simulink model "Comparison_between_Controllers_Ideal_PID_Form"  (R2018b)
settings: Solver=VariableStepAuto  StartTime=0.0  StopTime=500  FixedStep=1  RelTol=1e-3
undefined symbols (not defined in the file or in its folder): idss, s
libraries: cstblocks x29, simulink x14, peGeneralControl x4, slident x4, mpclib x3
(part 1 of 2)
settings Model: Creator=Trips  LastModifiedBy=Trips

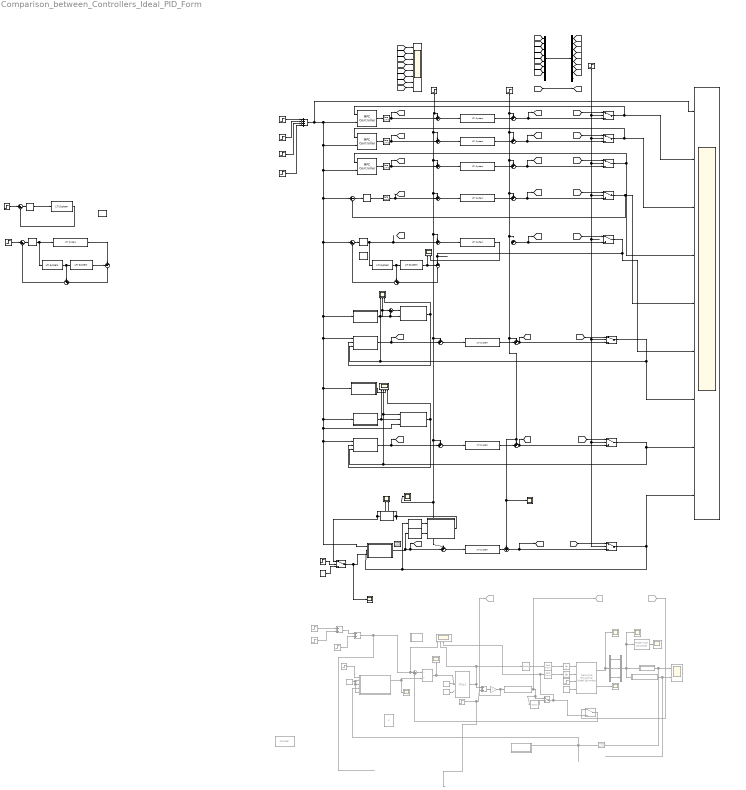
== system Comparison_between_Controllers_Ideal_PID_Form ==
  note: Winner Winner Chicken Dinner!
  note: MPC
  note: Testbedingungen: verändern der Totzeit und verändern der Verstärkung
  note: PI
  note: Smith Predictor
  note: Z
  note: Uncertainties
  note: Plant
  note: MRAC
  note: Z
  note: MIAC
  note: MRAC Better
  note: offset wegrechnen...
  Adaptive Mechanism : Subsystem
  Adaptive Mechanism1 : Subsystem
  Adaptive PI Controller : Subsystem  Commented=on
  Adaptive SmithPredictor : Subsystem
  Adaptive SmithPredictor1 : Subsystem
  Adaptive SmithPredictor2 : Subsystem
  Add{,1..9,11..12,16..17} (14 alike) : Sum  Inputs=++|
  Add10 : Sum  Inputs=++++
  Add13 : Sum  Commented=on
  Add14 : Sum  Commented=on
  Add15 : Sum  Commented=on
  Bus Creator2 : BusCreator  Commented=on  Inputs=3
  Bus Selector2 : BusSelector  Commented=on  OutputSignals=A,B,Ts
  Calculate DC Gain : Subsystem  Commented=on
  Calculate Time Constant : Subsystem  Commented=on
  Chien Hrones Reswick : Subsystem  Commented=on
  Constant1 : Constant  Value=0.5
  Constant6 : Constant  Commented=on  Value=0
  Demux : Demux  Outputs=8
  Divide1 : Product  Commented=on  Inputs=*/  OutMin=[1]  OutMax=[1]
  From24 : From  Commented=on  GotoTag=B8
  Gain1 : Gain  Commented=on
  Goto24 : Goto  Commented=on  GotoTag=U8
  Goto25 : Goto  Commented=on  GotoTag=A8
  Idmodel : slident/Models/Idmodel  Commented=on  sys=idss(-1,1,1,0,'Ts',1)  IC=0  noi=on  seed=[]
      settings: SourceProductName=System Identification Toolbox  SourceProductBaseCode=ID
  Kp_init : Constant  Commented=on
  Kp_init1 : Constant  Commented=on
  LTI System1 : cstblocks/LTI System  sys=0.5/(700*s+1)  IC=[]
  LTI System16 : cstblocks/LTI System  sys=0.5/(700*s+1)  IC=[]
  LTI System17 : cstblocks/LTI System  sys=exp(-s*600)  IC=[]
  LTI System2 : cstblocks/LTI System  sys=exp(-s*600)  IC=[]
  LTI System3 : cstblocks/LTI System  sys=0.5/(700*s+1)  IC=[]
  Low-Pass Filter (Discrete or Continuous) : peGeneralControl/Low-Pass Filter (Discrete or Continuous)  K=1  T=1200  B=inf  A=-inf  Ts=-1
  Low-Pass Filter (Discrete or Continuous)1 : peGeneralControl/Low-Pass Filter (Discrete or Continuous)  K=1  T=1200  B=inf  A=-inf  Ts=-1
  Low-Pass Filter (Discrete or Continuous)2 : peGeneralControl/Low-Pass Filter (Discrete or Continuous)  K=1  T=1200  B=inf  A=-inf  Ts=-1
  MPCFast_Robust : mpclib/MPC Controller  SCDEnableBlockLinearizationSpecification=on  mpcobj=mpc1_Faster_Robust  is_multiple=0  enable_value=0  return_u0=off  updateMPCinCallerWorkspace=on  md_inport=off  mv_inport=off  return_cost=off  return_mvseq=off  return_qpstatus=off  return_xseq=off  return_state=off  return_ovseq=off  state_inport=off  umin_inport=off  umax_inport=off  ymin_inport=off  ymax_inport=off  cc_inport=off  ywt_inport=off  uwt_inport=off  duwt_inport=off  rhoeps_inport=off  uref_inport=off  n_ts=70  n_p=15  n_mv=1  n_md=0  n_ud=0  n_mo=1  n_uo=0  BlockDataType=double  SampleTimeInherited=off  switch_inport=off
  MPCStandard : mpclib/MPC Controller  SCDEnableBlockLinearizationSpecification=on  mpcobj=mpc_Standard  is_multiple=0  enable_value=0  return_u0=off  updateMPCinCallerWorkspace=on  md_inport=off  mv_inport=off  return_cost=off  return_mvseq=off  return_qpstatus=off  return_xseq=off  return_state=off  return_ovseq=off  state_inport=off  umin_inport=off  umax_inport=off  ymin_inport=off  ymax_inport=off  cc_inport=off  ywt_inport=off  uwt_inport=off  duwt_inport=off  rhoeps_inport=off  uref_inport=off  n_ts=153  n_p=10  n_mv=1  n_md=0  n_ud=0  n_mo=1  n_uo=0  BlockDataType=double  SampleTimeInherited=off  switch_inport=off
  MPCStandardRobust : mpclib/MPC Controller  SCDEnableBlockLinearizationSpecification=on  mpcobj=mpc1_Standard_Robust  is_multiple=0  enable_value=0  return_u0=off  updateMPCinCallerWorkspace=on  md_inport=off  mv_inport=off  return_cost=off  return_mvseq=off  return_qpstatus=off  return_xseq=off  return_state=off  return_ovseq=off  state_inport=off  umin_inport=off  umax_inport=off  ymin_inport=off  ymax_inport=off  cc_inport=off  ywt_inport=off  uwt_inport=off  duwt_inport=off  rhoeps_inport=off  uref_inport=off  n_ts=153  n_p=10  n_mv=1  n_md=0  n_ud=0  n_mo=1  n_uo=0  BlockDataType=double  SampleTimeInherited=off  switch_inport=off
  Manual Switch : ManualSwitch  Commented=on
  Minus : Sum  Inputs=|+-
  Model Type Converter1 : slident/Estimators/Model Type Converter  Commented=on  InputModelType=ARX
      settings: SourceProductName=System Identification Toolbox  SourceProductBaseCode=ID
  Multiply : Product  Commented=on
  Mux : Mux  Inputs=8
  Outputs : Scope  NumInputPorts=9
  PID Controller : simulink/Continuous/PID Controller  Controller=PI  Form=Parallel  TimeDomain=Continuous-time  SampleTime=-1  IntegratorMethod=Forward Euler  FilterMethod=Forward Euler  ControllerParametersSource=internal  P=1.81017492228937  I=0.00195107565412744  D=118.272348286844  UseFilter=on  N=0.00420306193364532  TunerSelectOption=Transfer Function Based (PID Tuner App)  InitialConditionSource=internal  InitialConditionForIntegrator=0  InitialConditionForFilter=0  DifferentiatorICPrevScaledInput=0  ExternalReset=none  TrackingMode=off  Kt=1  LimitOutput=on  UpperSaturationLimit=100  LowerSaturationLimit=0  LinearizeAsGain=on  AntiWindupMode=none  Kb=1  POutMin=[]  POutMax=[]  IOutMin=[]  IOutMax=[]  DOutMin=[]  DOutMax=[]  NOutMin=[]  NOutMax=[]  SumOutMin=[]  SumOutMax=[]  SaturationOutMin=[]  SaturationOutMax=[]  PParamMin=[]  PParamMax=[]  IParamMin=[]  IParamMax=[]  DParamMin=[]  DParamMax=[]  NParamMin=[]  NParamMax=[]  KbParamMin=[]  KbParamMax=[]  KtParamMin=[]  KtParamMax=[]  KbOutMin=[]  KbOutMax=[]  KtOutMin=[]  KtOutMax=[]  IntegratorOutMin=[]  IntegratorOutMax=[]  FilterOutMin=[]  FilterOutMax=[]  SumI1OutMin=[]  SumI1OutMax=[]  SumI2OutMin=[]  SumI2OutMax=[]  SumI3OutMin=[]  SumI3OutMax=[]  SumI4OutMin=[]  SumI4OutMax=[]  SumDOutMin=[]  SumDOutMax=[]  DifferentiatorOutMin=[]  DifferentiatorOutMax=[]  FilterDiffOutCoefMin=[]  FilterDiffOutCoefMax=[]  ReciprocalOutMin=[]  ReciprocalOutMax=[]  SumDenOutMin=[]  SumDenOutMax=[]  SumNumOutMin=[]  SumNumOutMax=[]  DivideOutMin=[]  DivideOutMax=[]  IntegratorContinuousStateAttributes=''  IntegratorStateMustResolveToSignalObject=off  IntegratorRTWStateStorageClass=Auto  FilterContinuousStateAttributes=''  FilterStateMustResolveToSignalObject=off  FilterRTWStateStorageClass=Auto  ParallelPVariant=InternalParameters  IdealPVariant=Disabled  IVariant=InternalParameters  DVariant=Disabled  IntegratorVariant=Continuous  SatVariant=Enabled  AWVariant=Passthrough  PCopyVariant=Disabled  TRVariant=Disabled  FdbkBlocksVariant=Forward  IdealPFdbkVariant=Disabled  SatFdbkVariant=Disabled  DerivativeFilterVariant=Disabled  NVariant=Disabled  NCopyVariant=Disabled_SignalSpec  FilterICVariant=Disabled  IntegratorICVariant=InternalICs  ExternalResetVariant=Disabled  TRSumVariant=Passthrough  SumFdbkVariant=Disabled  SumVariant=Sum_PI
  PID Controller1 : simulink/Continuous/PID Controller  Controller=PI  Form=Parallel  TimeDomain=Continuous-time  SampleTime=-1  IntegratorMethod=Forward Euler  FilterMethod=Forward Euler  ControllerParametersSource=internal  P=2.08480938092905  I=0.0089383224092643  D=118.272348286844  UseFilter=on  N=0.00420306193364532  TunerSelectOption=Transfer Function Based (PID Tuner App)  InitialConditionSource=internal  InitialConditionForIntegrator=0  InitialConditionForFilter=0  DifferentiatorICPrevScaledInput=0  ExternalReset=none  TrackingMode=off  Kt=1  LimitOutput=on  UpperSaturationLimit=100  LowerSaturationLimit=0  LinearizeAsGain=on  AntiWindupMode=none  Kb=1  POutMin=[]  POutMax=[]  IOutMin=[]  IOutMax=[]  DOutMin=[]  DOutMax=[]  NOutMin=[]  NOutMax=[]  SumOutMin=[]  SumOutMax=[]  SaturationOutMin=[]  SaturationOutMax=[]  PParamMin=[]  PParamMax=[]  IParamMin=[]  IParamMax=[]  DParamMin=[]  DParamMax=[]  NParamMin=[]  NParamMax=[]  KbParamMin=[]  KbParamMax=[]  KtParamMin=[]  KtParamMax=[]  KbOutMin=[]  KbOutMax=[]  KtOutMin=[]  KtOutMax=[]  IntegratorOutMin=[]  IntegratorOutMax=[]  FilterOutMin=[]  FilterOutMax=[]  SumI1OutMin=[]  SumI1OutMax=[]  SumI2OutMin=[]  SumI2OutMax=[]  SumI3OutMin=[]  SumI3OutMax=[]  SumI4OutMin=[]  SumI4OutMax=[]  SumDOutMin=[]  SumDOutMax=[]  DifferentiatorOutMin=[]  DifferentiatorOutMax=[]  FilterDiffOutCoefMin=[]  FilterDiffOutCoefMax=[]  ReciprocalOutMin=[]  ReciprocalOutMax=[]  SumDenOutMin=[]  SumDenOutMax=[]  SumNumOutMin=[]  SumNumOutMax=[]  DivideOutMin=[]  DivideOutMax=[]  IntegratorContinuousStateAttributes=''  IntegratorStateMustResolveToSignalObject=off  IntegratorRTWStateStorageClass=Auto  FilterContinuousStateAttributes=''  FilterStateMustResolveToSignalObject=off  FilterRTWStateStorageClass=Auto  ParallelPVariant=InternalParameters  IdealPVariant=Disabled  IVariant=InternalParameters  DVariant=Disabled  IntegratorVariant=Continuous  SatVariant=Enabled  AWVariant=Passthrough  PCopyVariant=Disabled  TRVariant=Disabled  FdbkBlocksVariant=Forward  IdealPFdbkVariant=Disabled  SatFdbkVariant=Disabled  DerivativeFilterVariant=Disabled  NVariant=Disabled  NCopyVariant=Disabled_SignalSpec  FilterICVariant=Disabled  IntegratorICVariant=InternalICs  ExternalResetVariant=Disabled  TRSumVariant=Passthrough  SumFdbkVariant=Disabled  SumVariant=Sum_PI
  PID Controller2 : simulink/Continuous/PID Controller  Controller=PI  Form=Ideal  TimeDomain=Continuous-time  SampleTime=-1  IntegratorMethod=Forward Euler  FilterMethod=Forward Euler  ControllerParametersSource=internal  P=3.04732259067536  I=0.00445689106465138  D=118.272348286844  UseFilter=on  N=0.00420306193364532  TunerSelectOption=Transfer Function Based (PID Tuner App)  InitialConditionSource=internal  InitialConditionForIntegrator=0  InitialConditionForFilter=0  DifferentiatorICPrevScaledInput=0  ExternalReset=none  TrackingMode=off  Kt=1  LimitOutput=on  UpperSaturationLimit=100  LowerSaturationLimit=0  LinearizeAsGain=on  AntiWindupMode=none  Kb=1  POutMin=[]  POutMax=[]  IOutMin=[]  IOutMax=[]  DOutMin=[]  DOutMax=[]  NOutMin=[]  NOutMax=[]  SumOutMin=[]  SumOutMax=[]  SaturationOutMin=[]  SaturationOutMax=[]  PParamMin=[]  PParamMax=[]  IParamMin=[]  IParamMax=[]  DParamMin=[]  DParamMax=[]  NParamMin=[]  NParamMax=[]  KbParamMin=[]  KbParamMax=[]  KtParamMin=[]  KtParamMax=[]  KbOutMin=[]  KbOutMax=[]  KtOutMin=[]  KtOutMax=[]  IntegratorOutMin=[]  IntegratorOutMax=[]  FilterOutMin=[]  FilterOutMax=[]  SumI1OutMin=[]  SumI1OutMax=[]  SumI2OutMin=[]  SumI2OutMax=[]  SumI3OutMin=[]  SumI3OutMax=[]  SumI4OutMin=[]  SumI4OutMax=[]  SumDOutMin=[]  SumDOutMax=[]  DifferentiatorOutMin=[]  DifferentiatorOutMax=[]  FilterDiffOutCoefMin=[]  FilterDiffOutCoefMax=[]  ReciprocalOutMin=[]  ReciprocalOutMax=[]  SumDenOutMin=[]  SumDenOutMax=[]  SumNumOutMin=[]  SumNumOutMax=[]  DivideOutMin=[]  DivideOutMax=[]  IntegratorContinuousStateAttributes=''  IntegratorStateMustResolveToSignalObject=off  IntegratorRTWStateStorageClass=Auto  FilterContinuousStateAttributes=''  FilterStateMustResolveToSignalObject=off  FilterRTWStateStorageClass=Auto  ParallelPVariant=Passthrough  IdealPVariant=InternalParameters  IVariant=InternalParameters  DVariant=Disabled  IntegratorVariant=Continuous  SatVariant=Enabled  AWVariant=Passthrough  PCopyVariant=Disabled  TRVariant=Disabled  FdbkBlocksVariant=Forward  IdealPFdbkVariant=Disabled  SatFdbkVariant=Disabled  DerivativeFilterVariant=Disabled  NVariant=Disabled  NCopyVariant=Disabled_SignalSpec  FilterICVariant=Disabled  IntegratorICVariant=InternalICs  ExternalResetVariant=Disabled  TRSumVariant=Passthrough  SumFdbkVariant=Disabled  SumVariant=Sum_PI
  PID Controller3 : simulink/Continuous/PID Controller  Commented=on  Controller=PI  Form=Ideal  TimeDomain=Continuous-time  SampleTime=-1  IntegratorMethod=Forward Euler  FilterMethod=Forward Euler  ControllerParametersSource=internal  P=1.00442837242696  I=0.00143977155212025  D=0  UseFilter=on  N=100  TunerSelectOption=Transfer Function Based (PID Tuner App)  InitialConditionSource=internal  InitialConditionForIntegrator=0  InitialConditionForFilter=0  DifferentiatorICPrevScaledInput=0  ExternalReset=none  TrackingMode=off  Kt=1  LimitOutput=on  UpperSaturationLimit=100  LowerSaturationLimit=-100  LinearizeAsGain=on  AntiWindupMode=none  Kb=1  POutMin=[]  POutMax=[]  IOutMin=[]  IOutMax=[]  DOutMin=[]  DOutMax=[]  NOutMin=[]  NOutMax=[]  SumOutMin=[]  SumOutMax=[]  SaturationOutMin=[]  SaturationOutMax=[]  PParamMin=[]  PParamMax=[]  IParamMin=[]  IParamMax=[]  DParamMin=[]  DParamMax=[]  NParamMin=[]  NParamMax=[]  KbParamMin=[]  KbParamMax=[]  KtParamMin=[]  KtParamMax=[]  KbOutMin=[]  KbOutMax=[]  KtOutMin=[]  KtOutMax=[]  IntegratorOutMin=[]  IntegratorOutMax=[]  FilterOutMin=[]  FilterOutMax=[]  SumI1OutMin=[]  SumI1OutMax=[]  SumI2OutMin=[]  SumI2OutMax=[]  SumI3OutMin=[]  SumI3OutMax=[]  SumI4OutMin=[]  SumI4OutMax=[]  SumDOutMin=[]  SumDOutMax=[]  DifferentiatorOutMin=[]  DifferentiatorOutMax=[]  FilterDiffOutCoefMin=[]  FilterDiffOutCoefMax=[]  ReciprocalOutMin=[]  ReciprocalOutMax=[]  SumDenOutMin=[]  SumDenOutMax=[]  SumNumOutMin=[]  SumNumOutMax=[]  DivideOutMin=[]  DivideOutMax=[]  IntegratorContinuousStateAttributes=''  IntegratorStateMustResolveToSignalObject=off  IntegratorRTWStateStorageClass=Auto  FilterContinuousStateAttributes=''  FilterStateMustResolveToSignalObject=off  FilterRTWStateStorageClass=Auto  ParallelPVariant=Passthrough  IdealPVariant=InternalParameters  IVariant=InternalParameters  DVariant=Disabled  IntegratorVariant=Continuous  SatVariant=Enabled  AWVariant=Passthrough  PCopyVariant=Disabled  TRVariant=Disabled  FdbkBlocksVariant=Forward  IdealPFdbkVariant=Disabled  SatFdbkVariant=Disabled  DerivativeFilterVariant=Disabled  NVariant=Disabled  NCopyVariant=Disabled_SignalSpec  FilterICVariant=Disabled  IntegratorICVariant=InternalICs  ExternalResetVariant=Disabled  TRSumVariant=Passthrough  SumFdbkVariant=Disabled  SumVariant=Sum_PI
  PID Controller4 : simulink/Continuous/PID Controller  Controller=PID  Form=Parallel  TimeDomain=Continuous-time  SampleTime=-1  IntegratorMethod=Forward Euler  FilterMethod=Forward Euler  ControllerParametersSource=internal  P=1  I=1  D=0  UseFilter=on  N=100  TunerSelectOption=Transfer Function Based (PID Tuner App)  InitialConditionSource=internal  InitialConditionForIntegrator=0  InitialConditionForFilter=0  DifferentiatorICPrevScaledInput=0  ExternalReset=none  TrackingMode=off  Kt=1  LimitOutput=off  UpperSaturationLimit=inf  LowerSaturationLimit=-inf  LinearizeAsGain=on  AntiWindupMode=none  Kb=1  POutMin=[]  POutMax=[]  IOutMin=[]  IOutMax=[]  DOutMin=[]  DOutMax=[]  NOutMin=[]  NOutMax=[]  SumOutMin=[]  SumOutMax=[]  SaturationOutMin=[]  SaturationOutMax=[]  PParamMin=[]  PParamMax=[]  IParamMin=[]  IParamMax=[]  DParamMin=[]  DParamMax=[]  NParamMin=[]  NParamMax=[]  KbParamMin=[]  KbParamMax=[]  KtParamMin=[]  KtParamMax=[]  KbOutMin=[]  KbOutMax=[]  KtOutMin=[]  KtOutMax=[]  IntegratorOutMin=[]  IntegratorOutMax=[]  FilterOutMin=[]  FilterOutMax=[]  SumI1OutMin=[]  SumI1OutMax=[]  SumI2OutMin=[]  SumI2OutMax=[]  SumI3OutMin=[]  SumI3OutMax=[]  SumI4OutMin=[]  SumI4OutMax=[]  SumDOutMin=[]  SumDOutMax=[]  DifferentiatorOutMin=[]  DifferentiatorOutMax=[]  FilterDiffOutCoefMin=[]  FilterDiffOutCoefMax=[]  ReciprocalOutMin=[]  ReciprocalOutMax=[]  SumDenOutMin=[]  SumDenOutMax=[]  SumNumOutMin=[]  SumNumOutMax=[]  DivideOutMin=[]  DivideOutMax=[]  IntegratorContinuousStateAttributes=''  IntegratorStateMustResolveToSignalObject=off  IntegratorRTWStateStorageClass=Auto  FilterContinuousStateAttributes=''  FilterStateMustResolveToSignalObject=off  FilterRTWStateStorageClass=Auto  ParallelPVariant=InternalParameters  IdealPVariant=Disabled  IVariant=InternalParameters  DVariant=InternalParameters  IntegratorVariant=Continuous  SatVariant=Disabled  AWVariant=Passthrough  PCopyVariant=Disabled  TRVariant=Disabled  FdbkBlocksVariant=Forward  IdealPFdbkVariant=Disabled  SatFdbkVariant=Disabled  DerivativeFilterVariant=ContFilter  NVariant=InternalParameters  NCopyVariant=Disabled  FilterICVariant=InternalICsFilter  IntegratorICVariant=InternalICs  ExternalResetVariant=Disabled  TRSumVariant=Passthrough  SumFdbkVariant=Disabled  SumVariant=Sum_PID
  PID Controller5 : simulink/Continuous/PID Controller  Controller=PI  Form=Parallel  TimeDomain=Continuous-time  SampleTime=-1  IntegratorMethod=Forward Euler  FilterMethod=Forward Euler  ControllerParametersSource=internal  P=3.04732259067536  I=0.00445689106465138  D=118.272348286844  UseFilter=on  N=0.00420306193364532  TunerSelectOption=Transfer Function Based (PID Tuner App)  InitialConditionSource=internal  InitialConditionForIntegrator=0  InitialConditionForFilter=0  DifferentiatorICPrevScaledInput=0  ExternalReset=none  TrackingMode=off  Kt=1  LimitOutput=on  UpperSaturationLimit=100  LowerSaturationLimit=0  LinearizeAsGain=on  AntiWindupMode=none  Kb=1  POutMin=[]  POutMax=[]  IOutMin=[]  IOutMax=[]  DOutMin=[]  DOutMax=[]  NOutMin=[]  NOutMax=[]  SumOutMin=[]  SumOutMax=[]  SaturationOutMin=[]  SaturationOutMax=[]  PParamMin=[]  PParamMax=[]  IParamMin=[]  IParamMax=[]  DParamMin=[]  DParamMax=[]  NParamMin=[]  NParamMax=[]  KbParamMin=[]  KbParamMax=[]  KtParamMin=[]  KtParamMax=[]  KbOutMin=[]  KbOutMax=[]  KtOutMin=[]  KtOutMax=[]  IntegratorOutMin=[]  IntegratorOutMax=[]  FilterOutMin=[]  FilterOutMax=[]  SumI1OutMin=[]  SumI1OutMax=[]  SumI2OutMin=[]  SumI2OutMax=[]  SumI3OutMin=[]  SumI3OutMax=[]  SumI4OutMin=[]  SumI4OutMax=[]  SumDOutMin=[]  SumDOutMax=[]  DifferentiatorOutMin=[]  DifferentiatorOutMax=[]  FilterDiffOutCoefMin=[]  FilterDiffOutCoefMax=[]  ReciprocalOutMin=[]  ReciprocalOutMax=[]  SumDenOutMin=[]  SumDenOutMax=[]  SumNumOutMin=[]  SumNumOutMax=[]  DivideOutMin=[]  DivideOutMax=[]  IntegratorContinuousStateAttributes=''  IntegratorStateMustResolveToSignalObject=off  IntegratorRTWStateStorageClass=Auto  FilterContinuousStateAttributes=''  FilterStateMustResolveToSignalObject=off  FilterRTWStateStorageClass=Auto  ParallelPVariant=InternalParameters  IdealPVariant=Disabled  IVariant=InternalParameters  DVariant=Disabled  IntegratorVariant=Continuous  SatVariant=Enabled  AWVariant=Passthrough  PCopyVariant=Disabled  TRVariant=Disabled  FdbkBlocksVariant=Forward  IdealPFdbkVariant=Disabled  SatFdbkVariant=Disabled  DerivativeFilterVariant=Disabled  NVariant=Disabled  NCopyVariant=Disabled_SignalSpec  FilterICVariant=Disabled  IntegratorICVariant=InternalICs  ExternalResetVariant=Disabled  TRSumVariant=Passthrough  SumFdbkVariant=Disabled  SumVariant=Sum_PI
  PID Controller6 : simulink/Continuous/PID Controller  Controller=PI  Form=Parallel  TimeDomain=Continuous-time  SampleTime=-1  IntegratorMethod=Forward Euler  FilterMethod=Forward Euler  ControllerParametersSource=internal  P=1  I=1  D=0  UseFilter=on  N=100  TunerSelectOption=Transfer Function Based (PID Tuner App)  InitialConditionSource=internal  InitialConditionForIntegrator=0  InitialConditionForFilter=0  DifferentiatorICPrevScaledInput=0  ExternalReset=none  TrackingMode=off  Kt=1  LimitOutput=off  UpperSaturationLimit=inf  LowerSaturationLimit=-inf  LinearizeAsGain=on  AntiWindupMode=none  Kb=1  POutMin=[]  POutMax=[]  IOutMin=[]  IOutMax=[]  DOutMin=[]  DOutMax=[]  NOutMin=[]  NOutMax=[]  SumOutMin=[]  SumOutMax=[]  SaturationOutMin=[]  SaturationOutMax=[]  PParamMin=[]  PParamMax=[]  IParamMin=[]  IParamMax=[]  DParamMin=[]  DParamMax=[]  NParamMin=[]  NParamMax=[]  KbParamMin=[]  KbParamMax=[]  KtParamMin=[]  KtParamMax=[]  KbOutMin=[]  KbOutMax=[]  KtOutMin=[]  KtOutMax=[]  IntegratorOutMin=[]  IntegratorOutMax=[]  FilterOutMin=[]  FilterOutMax=[]  SumI1OutMin=[]  SumI1OutMax=[]  SumI2OutMin=[]  SumI2OutMax=[]  SumI3OutMin=[]  SumI3OutMax=[]  SumI4OutMin=[]  SumI4OutMax=[]  SumDOutMin=[]  SumDOutMax=[]  DifferentiatorOutMin=[]  DifferentiatorOutMax=[]  FilterDiffOutCoefMin=[]  FilterDiffOutCoefMax=[]  ReciprocalOutMin=[]  ReciprocalOutMax=[]  SumDenOutMin=[]  SumDenOutMax=[]  SumNumOutMin=[]  SumNumOutMax=[]  DivideOutMin=[]  DivideOutMax=[]  IntegratorContinuousStateAttributes=''  IntegratorStateMustResolveToSignalObject=off  IntegratorRTWStateStorageClass=Auto  FilterContinuousStateAttributes=''  FilterStateMustResolveToSignalObject=off  FilterRTWStateStorageClass=Auto  ParallelPVariant=InternalParameters  IdealPVariant=Disabled  IVariant=InternalParameters  DVariant=Disabled  IntegratorVariant=Continuous  SatVariant=Disabled  AWVariant=Passthrough  PCopyVariant=Disabled  TRVariant=Disabled  FdbkBlocksVariant=Forward  IdealPFdbkVariant=Disabled  SatFdbkVariant=Disabled  DerivativeFilterVariant=Disabled  NVariant=Disabled  NCopyVariant=Disabled_SignalSpec  FilterICVariant=Disabled  IntegratorICVariant=InternalICs  ExternalResetVariant=Disabled  TRSumVariant=Passthrough  SumFdbkVariant=Disabled  SumVariant=Sum_PI
  Plant{,1..7,9} (9 alike) : cstblocks/LTI System  sys=0.5/(700*s+1)*exp(-s*600)  IC=[]
  Plant8 : cstblocks/LTI System  Commented=on  sys=0.5/(700*s+1)*exp(-s*600)  IC=[]
  Rate Limiter{1..2,4..6} (5 alike) : RateLimiter  RisingSlewLimit=0.05  FallingSlewLimit=-0.05  SampleTimeMode=inherited
  Rate Limiter3 : RateLimiter  Commented=on  SampleTimeMode=inherited
  Rate Transition : RateTransition  Commented=on  OutPortSampleTime=10
  Rate Transition1 : RateTransition  Commented=on  OutPortSampleTime=10
  Recursive Polynomial Model Estimator1 : slident/Estimators/Recursive Polynomial Model Estimator  Commented=on  ModelStructure=ARX  InitialEstimateSource=None  A0=1  B0=1  C0=1  D0=1  F0=1  nk=1  P0=1  InitialInputs=0  InitialOutputs=0  History=Infinite  WindowLength=6000  EstimationMethod=Kalman Filter  AdaptationParameter=0.1  HasTimeVaryingAdaptationParameter=off  NormalizationBias=eps  OutputError=on  OutputP=off  AddEnablePort=on  ExternalReset=Rising  InputProcessing=Sample-based  Ts=10
      settings: SourceProductName=System Identification Toolbox  SourceProductBaseCode=ID
  Reference_Model : Subsystem
  Reference_Model1 : Subsystem
  Reference_Model2 : Subsystem
  References : Step
  References1 : Step  Time=12000  After=2
  References2 : Step  Time=18000  After=3
  References3 : Step  Time=35000  After=3
  Scope : Scope  NumInputPorts=8
  Scope1 : Scope  NumInputPorts=2
  Scope10 : Scope  Commented=on  NumInputPorts=2
  Scope{5,7..9,11..12} (6 alike) : Scope  Commented=on
  Scope13 : Scope
  Scope14 : Scope
  Scope15 : Scope
  Scope2 : Scope  NumInputPorts=2
  Scope3 : Scope  NumInputPorts=4
  Scope4 : Scope  NumInputPorts=3
  Scope6 : Scope  Commented=on  NumInputPorts=5
  Starte adaption : Step  Commented=on  Time=0  SampleTime=1
  Step : Step  Time=0  SampleTime=1
  Step1 : Step  Time=4000  After=0  SampleTime=0
  Step10 : Step  SampleTime=0
  Step2 : Step  Time=4000  SampleTime=0
  Step3 : Step  Time=7000  After=0  SampleTime=0
  Step4 : Step  Commented=on  Time=4000  SampleTime=0.1
  Step5 : Step  Commented=on  Time=10000  After=2  SampleTime=0.1
  Step6 : Step  Commented=on  Time=6000  After=-1  SampleTime=0.1
  Step7 : Step  Commented=on  Time=15  After=3  SampleTime=0.1
  Step8 : Step  Commented=on  Time=14000  After=-5  SampleTime=0.1
  Step9 : Step  SampleTime=0
  Subsystem : Subsystem  Commented=on
  Subtract : Sum  Commented=on  Inputs=|+-
  Sum{1,5,18..19} (4 alike) : Sum  Inputs=++|
  Sum{2..3,6,16} (4 alike) : Sum  Inputs=|+-
  Sum17 : Sum  Inputs=-+|
  Sum4 : Sum  Inputs=-+|
  Switch{,1..8} (9 alike) : Switch  Criteria=u2 > Threshold
  Switch9 : Switch  Commented=on  Criteria=u2 > Threshold
  System Identification : Subsystem
  Ti_init : Constant  Commented=on
  Transport Delay : TransportDelay  Commented=on
  Transport Delay1 : TransportDelay  Commented=on  DelayTime=600
  Unit Delay4 : UnitDelay  Commented=on  InitialCondition=[0]  SampleTime=10
  Unit Delay5 : UnitDelay  Commented=on  SampleTime=10
  wires:
  MPCStandard/1 -> Rate Limiter5/1  "MPCStandard"
  Add2/1 -> Plant/1
  Switch/1 -> MPCStandard/1, Outputs/2  "MPCStandard"
  PID Controller/1 -> Rate Limiter2/1  "PID"
  Minus/1 -> PID Controller/1
  Switch3/1 -> Outputs/5, Minus/2  "PID"
  Add1/1 -> Plant1/1
  MPCStandardRobust/1 -> Rate Limiter4/1  "MPCStandardRobust"
  Switch1/1 -> MPCStandardRobust/1, Outputs/3  "MPCStandardRobust"
  Add3/1 -> Plant2/1
  MPCFast_Robust/1 -> Rate Limiter1/1  "MPCFast_Robust"
  Switch2/1 -> MPCFast_Robust/1, Outputs/4  "MPCFast_Robust"
  Add4/1 -> Plant3/1
  Sum17/1 -> Sum18/2
  LTI System16/1 -> LTI System17/1, Sum18/1
  Sum18/1 -> Sum16/2
  LTI System17/1 -> Sum17/1, Scope1/1
  PID Controller2/1 -> Plant4/1, LTI System16/1  "SmithPredictor"
  Sum16/1 -> PID Controller2/1
  Sum19/1 -> ?  "smith"
  Add7/1 -> [A1], Switch/3  "MPCStandard"
  Add8/1 -> Switch1/3, [A2]  "MPCStandardRobust"
  Add9/1 -> Switch2/3, [A3]  "MPCFast_Robust"
  Add6/1 -> Switch3/3, [A4]  "PID"
  Sum1/1 -> Switch4/3, [A5]  "SmithPredictor"
  Demux/3 -> [B3]
  Demux/2 -> [B2]
  Demux/1 -> [B1]
  Switch4/1 -> Outputs/6, Scope1/2  "SmithPredictor"
  Rate Limiter1/1 -> [U3], Add4/2
  Reference_Model/1(Ym) -> Scope4/1, Adaptive Mechanism/2(Ym), Sum2/2  "Reference Model"
  Add5/1 -> [A6], Switch5/3
  Adaptive SmithPredictor/1(U) -> [U6], Add/2  "Adaptive"
  Adaptive Mechanism/1(theta) -> Scope4/3, Adaptive SmithPredictor/2(theta)  "theta"
  Add/1 -> Plant5/1
  Sum2/1 -> Adaptive Mechanism/1(e)  "e"
  Switch5/1 -> Adaptive SmithPredictor/3(Yp), Scope4/2, Sum2/1, Outputs/7  "MRAC_SmithPredictor"
  [B6] -> Switch5/1
  [A1] -> Mux/1
  [A2] -> Mux/2
  [A3] -> Mux/3
  [A4] -> Mux/4
  [A5] -> Mux/5
  [A6] -> Mux/6
  Demux/6 -> [B6]
  Demux/4 -> [B4]
  Demux/5 -> [B5]
  [B1] -> Switch/1
  [B2] -> Switch1/1
  [B3] -> Switch2/1
  [B4] -> Switch3/1
  [B5] -> Switch4/1
  [U1] -> Scope/1
  [U2] -> Scope/2
  [U3] -> Scope/3
  [U4] -> Scope/4
  [U5] -> Scope/5
  [U6] -> Scope/6
  Switch8/1 -> Adaptive SmithPredictor2/3(Yp), Scope3/2, Adaptive Mechanism1/1(Yreal), Outputs/8  "MRAC_SmithPredictorBetter"
  [U7] -> Scope/7
  [A7] -> Mux/7
  Demux/7 -> [B7]
  Constant1/1 -> Switch6/3
  Step2/1 -> Switch6/2
  Plant5/1 -> Add5/2
  Plant4/1 -> Sum17/2  "SmithPredictor"
  Plant1/1 -> Add6/2  "PID"
  Plant3/1 -> Add9/2  "MPCFast_Robust"
  Plant2/1 -> Add8/2  "MPCStandardRobust"
  Plant/1 -> Add7/2  "MPCStandard"
  References/1 -> Add10/1  "r"
  References1/1 -> Add10/2  "r"
  Rate Limiter2/1 -> Add1/2, [U4]
  Rate Limiter4/1 -> [U2], Add3/2
  Rate Limiter5/1 -> [U1], Add2/2
  Switch7/1 -> Low-Pass Filter (Discrete or Continuous)1/1, Adaptive SmithPredictor1/2(Yp), Outputs/9  "MIAC_SmithPredictor"
  Adaptive SmithPredictor1/1(U) -> Low-Pass Filter (Discrete or Continuous)2/1, Add16/2, [U8]  "Adaptive"
  Switch6/1 -> Scope13/1, Adaptive SmithPredictor1/3(EstimatedGain)
  Step3/1 -> Add7/1, Scope15/1, Add17/1, Add12/1, Add5/1, Add6/1, Add9/1, Add8/1
  Reference_Model1/1(Ym) -> Adaptive Mechanism1/2(Ym), Scope3/1  "Reference Model"
  Plant6/1 -> Add12/2
  Step1/1 -> Add2/1, Sum19/1, Add11/1, Scope14/1, Add16/1, Add/1, Add1/1, Add4/1, Add3/1
  Add11/1 -> Plant6/1
  Adaptive Mechanism1/1(theta) -> Scope3/4, Adaptive SmithPredictor2/2(theta)  "theta"
  Step/1 -> Switch2/2, Switch3/2, Switch7/2, Switch8/2, Switch5/2, Switch1/2, Switch/2
  Adaptive SmithPredictor2/1(U) -> [U7], Add11/2  "Adaptive"
  Reference_Model2/1(Ym) -> Scope3/3  "Reference Model"
  References2/1 -> Add10/3  "r"
  Divide1/1 -> PID Controller3/1, Scope12/1  "output"
  Subtract/1 -> Divide1/1  "e"
  Rate Transition1/1 -> Unit Delay5/1
  Gain1/1 -> Goto24/1, Plant8/1
  Transport Delay1/1 -> Rate Transition/1
  ? -> Scope6/5  "u non adaptive"
  Plant8/1 -> Goto25/1, Transport Delay/1, Manual Switch/1  "y"
  Step8/1 -> Add15/2  "u"
  Step4/1 -> Subsystem/1(Start)  "u"
  Calculate Time Constant/1("OutTimeConstant ") -> Scope10/2
  ? -> Chien Hrones Reswick/3(Td)
  Model Type Converter1/1 -> Scope8/1
  Add15/1 -> Gain1/1
  ? -> Scope6/4  "non adaptive"
  Kp_init/1 -> ?
  Manual Switch/1 -> Switch9/3, Rate Transition1/1, Scope6/3  "Adaptive"
  Kp_init1/1 -> Subsystem/2(KP_init), Subsystem/3(Ti_init), Subsystem/5(Ti_estimated)
  PID Controller3/1 -> Transport Delay1/1, Scope6/2, Add15/1  "u adaptive"
  Step6/1 -> Add13/1
  Add14/1 -> Scope6/1, Subtract/1  "w"
  Step5/1 -> Add13/2
  Bus Selector2/3 -> Bus Creator2/3  "<Ts>"
  ? -> Chien Hrones Reswick/2(T)  "limited time constant"
  Starte adaption/1 -> Recursive Polynomial Model Estimator1/3
  Bus Creator2/1 -> Calculate Time Constant/1(Params), Calculate DC Gain/1(Params), Scope9/1, Model Type Converter1/1
  Transport Delay/1 -> Manual Switch/2
  Step7/1 -> Add14/2
  Constant6/1 -> Recursive Polynomial Model Estimator1/4
  Ti_init/1 -> ?
  Recursive Polynomial Model Estimator1/1 -> Scope5/1, Bus Selector2/1
  Calculate DC Gain/1(DCGain) -> Scope10/1, Rate Limiter3/1
  Rate Transition/1 -> Unit Delay4/1
  Bus Selector2/1 -> Bus Creator2/1  "<A>"
  Unit Delay5/1 -> Recursive Polynomial Model Estimator1/2  "output"
  Add13/1 -> Add14/1  "w"
  Recursive Polynomial Model Estimator1/2 -> Scope7/1
  Rate Limiter3/1 -> Subsystem/4(Kp_estimated), Chien Hrones Reswick/1(K)  "limited Gain"
  Bus Selector2/2 -> Bus Creator2/2  "<B>"
  Unit Delay4/1 -> Recursive Polynomial Model Estimator1/1  "input"
  Subsystem/1(Kp) -> Divide1/2, Scope11/1  "P"
  [U8] -> Scope/8
  ? -> Mux/8
  Demux/8 -> ?
  From24/1 -> Switch9/1
  Switch9/1 -> Subtract/2  "Adaptive_SmithPredictor"
  Add12/1 -> [A7], Switch8/3
  [B7] -> Switch8/1
  [A8] -> [B8]
  Mux/1 -> Demux/1
  Add17/1 -> [A8], Switch7/3
  [B8] -> Switch7/1
  System Identification/1(Gain) -> Scope2/2, Low-Pass Filter (Discrete or Continuous)/1
  Add16/1 -> Plant7/1
  Low-Pass Filter (Discrete or Continuous)/1 -> Switch6/1, Scope2/1
  Low-Pass Filter (Discrete or Continuous)1/1 -> System Identification/1(Output)
  Low-Pass Filter (Discrete or Continuous)2/1 -> System Identification/2(Input)
  Plant7/1 -> Add17/2
  References3/1 -> Add10/4  "r"
  Plant9/1 -> Sum4/2  "SmithPredictor"
  PID Controller4/1 -> Plant9/1, LTI System1/1  "SmithPredictor"
  LTI System2/1 -> Sum4/1
  Sum4/1 -> Sum5/2
  LTI System1/1 -> LTI System2/1, Sum5/1
  Add10/1 -> Outputs/1, MPCStandardRobust/2, MPCFast_Robust/2, Reference_Model/1(r), Reference_Model2/1(r), Reference_Model1/1(r), Adaptive Mechanism1/3(setpoint), Adaptive SmithPredictor1/1(r), Adaptive SmithPredictor2/1(r), Adaptive SmithPredictor/1(r), Sum16/1, Minus/1, MPCStandard/2  "setpoint"
  Sum5/1 -> Sum3/2
  Sum3/1 -> PID Controller4/1
  Step9/1 -> Sum3/1
  PID Controller6/1 -> LTI System3/1  "SmithPredictor"
  LTI System3/1 -> Sum6/2
  Step10/1 -> Sum6/1
  Sum6/1 -> PID Controller6/1

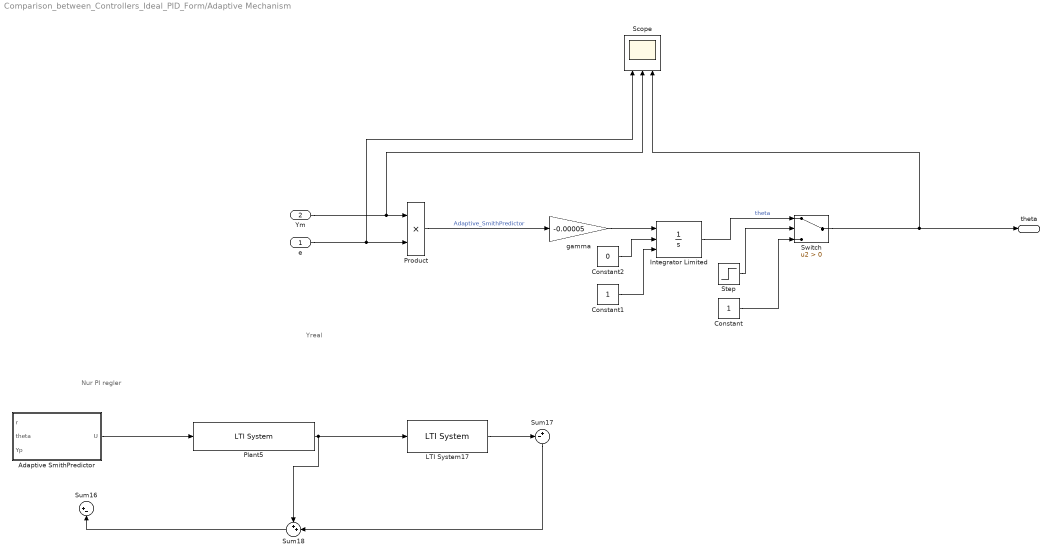
== system Comparison_between_Controllers_Ideal_PID_Form/Adaptive Mechanism ==
  note: Nur PI regler
  note: Yreal
  e : Inport
  Ym : Inport  Port=2
  Adaptive SmithPredictor : Subsystem
  Constant : Constant
  Constant1 : Constant
  Constant2 : Constant  Value=0
  Integrator Limited : Integrator  ExternalReset=rising  InitialConditionSource=external  InitialCondition=1  LimitOutput=on  UpperSaturationLimit=100  LowerSaturationLimit=-100
  LTI System17 : cstblocks/LTI System  sys=exp(-s*600)  IC=[]
  Plant5 : cstblocks/LTI System  sys=0.5/(700*s+1)  IC=[]
  Product : Product
  Scope : Scope  NumInputPorts=3
  Step : Step  Time=0  SampleTime=0
  Sum16 : Sum  Inputs=|+-
  Sum17 : Sum  Inputs=-+|
  Sum18 : Sum  Inputs=++|
  Switch : Switch  Criteria=u2 > Threshold
  gamma : Gain  Gain=-0.00005
  theta : Outport
  wires:
  Ym/1 -> Scope/2, Product/1
  e/1 -> Scope/1, Product/2
  gamma/1 -> Integrator Limited/1
  Integrator Limited/1 -> Switch/1  "theta"
  Constant/1 -> Switch/3
  Step/1 -> Switch/2
  Constant1/1 -> Integrator Limited/3
  Constant2/1 -> Integrator Limited/2
  Product/1 -> gamma/1  "Adaptive_SmithPredictor"
  Sum18/1 -> Sum16/2
  Plant5/1 -> LTI System17/1, Sum18/1
  Sum17/1 -> Sum18/2
  LTI System17/1 -> Sum17/1
  Adaptive SmithPredictor/1(U) -> Plant5/1
  ? -> Sum17/2
  Switch/1 -> theta/1, Scope/3

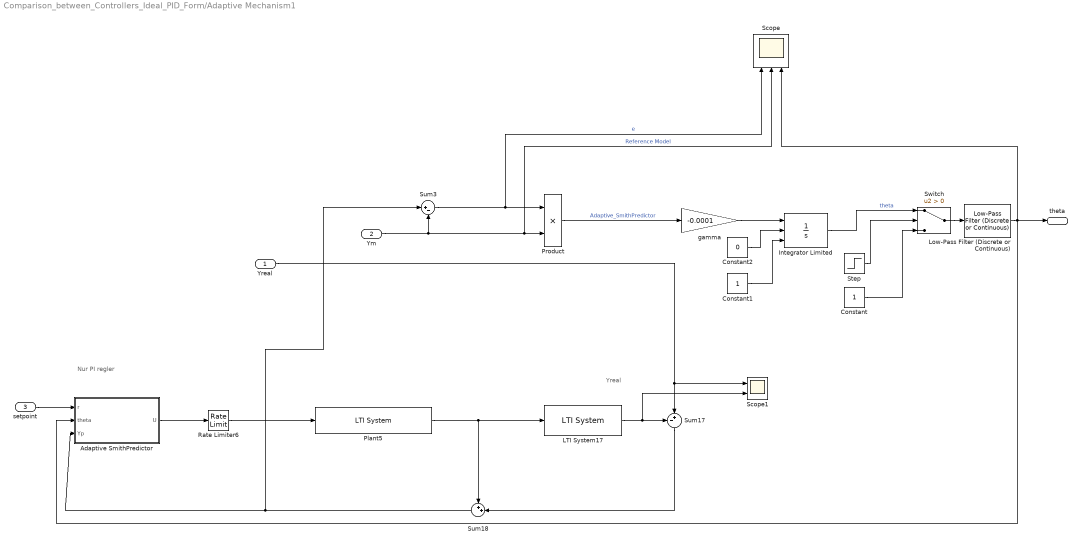
== system Comparison_between_Controllers_Ideal_PID_Form/Adaptive Mechanism1 ==
  note: Nur PI regler
  note: Yreal
  Yreal : Inport
  Ym : Inport  Port=2
  setpoint : Inport  Port=3
  Adaptive SmithPredictor : Subsystem
  Constant : Constant
  Constant1 : Constant
  Constant2 : Constant  Value=0
  Integrator Limited : Integrator  ExternalReset=rising  InitialConditionSource=external  InitialCondition=1  LimitOutput=on  UpperSaturationLimit=100  LowerSaturationLimit=-100
  LTI System17 : cstblocks/LTI System  sys=exp(-s*600)  IC=[]
  Low-Pass Filter (Discrete or Continuous) : peGeneralControl/Low-Pass Filter (Discrete or Continuous)  K=1  T=1200  B=inf  A=-inf  Ts=-1
  Plant5 : cstblocks/LTI System  sys=0.5/(700*s+1)  IC=[]
  Product : Product
  Rate Limiter6 : RateLimiter  RisingSlewLimit=0.05  FallingSlewLimit=-0.05  SampleTimeMode=inherited
  Scope : Scope  NumInputPorts=3
  Scope1 : Scope  NumInputPorts=2
  Step : Step  Time=0  SampleTime=0
  Sum17 : Sum  Inputs=-+|
  Sum18 : Sum  Inputs=++|
  Sum3 : Sum  Inputs=|+-
  Switch : Switch  Criteria=u2 > Threshold
  gamma : Gain  Gain=-0.0001
  theta : Outport
  wires:
  Switch/1 -> Low-Pass Filter (Discrete or Continuous)/1
  gamma/1 -> Integrator Limited/1
  Integrator Limited/1 -> Switch/1  "theta"
  Constant/1 -> Switch/3
  Step/1 -> Switch/2
  Constant1/1 -> Integrator Limited/3
  Constant2/1 -> Integrator Limited/2
  Product/1 -> gamma/1  "Adaptive_SmithPredictor"
  Plant5/1 -> LTI System17/1, Sum18/1
  Sum17/1 -> Sum18/2
  LTI System17/1 -> Scope1/2, Sum17/1
  Adaptive SmithPredictor/1(U) -> Rate Limiter6/1
  Ym/1 -> Sum3/2, Scope/2, Product/2  "Reference Model"
  Sum3/1 -> Scope/1, Product/1  "e"
  Yreal/1 -> Sum17/2, Scope1/1
  setpoint/1 -> Adaptive SmithPredictor/1(r)
  Sum18/1 -> Sum3/1, Adaptive SmithPredictor/3(Yp)
  Rate Limiter6/1 -> Plant5/1
  Low-Pass Filter (Discrete or Continuous)/1 -> Adaptive SmithPredictor/2(theta), Scope/3, theta/1

== system Comparison_between_Controllers_Ideal_PID_Form/Adaptive PI Controller ==
  DC Gain : Inport
  e : Inport  Port=2
  Divide1 : Product  Inputs=*/
  e_Adapted : Outport
  wires:
  e/1 -> Divide1/1
  Divide1/1 -> e_Adapted/1
  DC Gain/1 -> Divide1/2

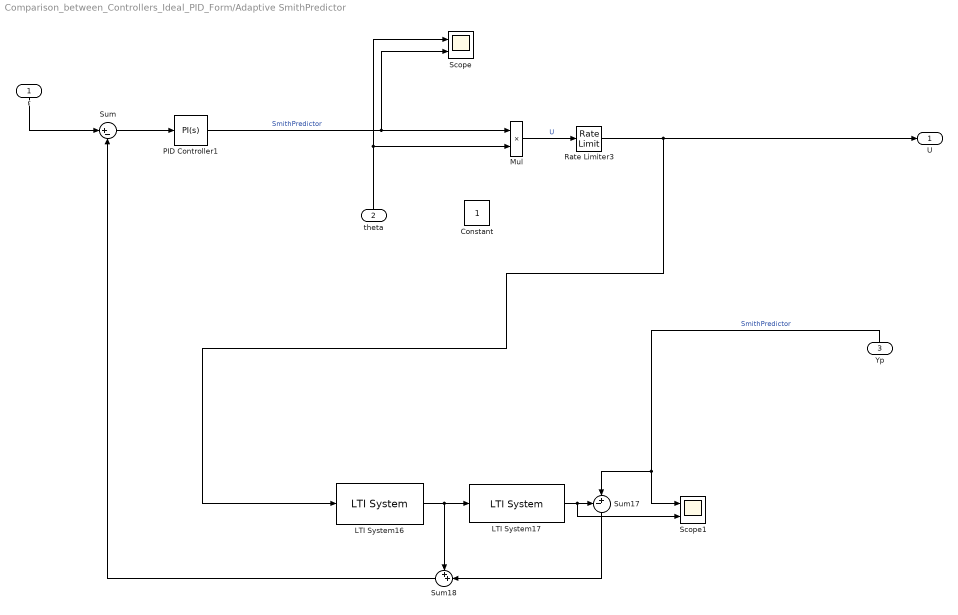
== system Comparison_between_Controllers_Ideal_PID_Form/Adaptive SmithPredictor ==
  r : Inport
  theta : Inport  Port=2
  Yp : Inport  Port=3
  Constant : Constant
  LTI System16 : cstblocks/LTI System  sys=0.5/(700*s+1)  IC=[]
  LTI System17 : cstblocks/LTI System  sys=exp(-s*600)  IC=[]
  Mul : Product
  PID Controller1 : simulink/Continuous/PID Controller  Controller=PI  Form=Parallel  TimeDomain=Continuous-time  SampleTime=-1  IntegratorMethod=Forward Euler  FilterMethod=Forward Euler  ControllerParametersSource=internal  P=3.04732259067536  I=0.00445689106465138  D=118.272348286844  UseFilter=on  N=0.00420306193364532  TunerSelectOption=Transfer Function Based (PID Tuner App)  InitialConditionSource=internal  InitialConditionForIntegrator=0  InitialConditionForFilter=0  DifferentiatorICPrevScaledInput=0  ExternalReset=none  TrackingMode=off  Kt=1  LimitOutput=on  UpperSaturationLimit=100  LowerSaturationLimit=0  LinearizeAsGain=on  AntiWindupMode=none  Kb=1  POutMin=[]  POutMax=[]  IOutMin=[]  IOutMax=[]  DOutMin=[]  DOutMax=[]  NOutMin=[]  NOutMax=[]  SumOutMin=[]  SumOutMax=[]  SaturationOutMin=[]  SaturationOutMax=[]  PParamMin=[]  PParamMax=[]  IParamMin=[]  IParamMax=[]  DParamMin=[]  DParamMax=[]  NParamMin=[]  NParamMax=[]  KbParamMin=[]  KbParamMax=[]  KtParamMin=[]  KtParamMax=[]  KbOutMin=[]  KbOutMax=[]  KtOutMin=[]  KtOutMax=[]  IntegratorOutMin=[]  IntegratorOutMax=[]  FilterOutMin=[]  FilterOutMax=[]  SumI1OutMin=[]  SumI1OutMax=[]  SumI2OutMin=[]  SumI2OutMax=[]  SumI3OutMin=[]  SumI3OutMax=[]  SumI4OutMin=[]  SumI4OutMax=[]  SumDOutMin=[]  SumDOutMax=[]  DifferentiatorOutMin=[]  DifferentiatorOutMax=[]  FilterDiffOutCoefMin=[]  FilterDiffOutCoefMax=[]  ReciprocalOutMin=[]  ReciprocalOutMax=[]  SumDenOutMin=[]  SumDenOutMax=[]  SumNumOutMin=[]  SumNumOutMax=[]  DivideOutMin=[]  DivideOutMax=[]  IntegratorContinuousStateAttributes=''  IntegratorStateMustResolveToSignalObject=off  IntegratorRTWStateStorageClass=Auto  FilterContinuousStateAttributes=''  FilterStateMustResolveToSignalObject=off  FilterRTWStateStorageClass=Auto  ParallelPVariant=InternalParameters  IdealPVariant=Disabled  IVariant=InternalParameters  DVariant=Disabled  IntegratorVariant=Continuous  SatVariant=Enabled  AWVariant=Passthrough  PCopyVariant=Disabled  TRVariant=Disabled  FdbkBlocksVariant=Forward  IdealPFdbkVariant=Disabled  SatFdbkVariant=Disabled  DerivativeFilterVariant=Disabled  NVariant=Disabled  NCopyVariant=Disabled_SignalSpec  FilterICVariant=Disabled  IntegratorICVariant=InternalICs  ExternalResetVariant=Disabled  TRSumVariant=Passthrough  SumFdbkVariant=Disabled  SumVariant=Sum_PI
  Rate Limiter3 : RateLimiter  RisingSlewLimit=0.05  FallingSlewLimit=-0.05  SampleTimeMode=inherited
  Scope : Scope  NumInputPorts=2
  Scope1 : Scope  NumInputPorts=2
  Sum : Sum  Inputs=|+-
  Sum17 : Sum  Inputs=-+|
  Sum18 : Sum  Inputs=++|
  U : Outport
  wires:
  r/1 -> Sum/1
  Sum/1 -> PID Controller1/1
  Mul/1 -> Rate Limiter3/1  "U"
  PID Controller1/1 -> Scope/2, Mul/1  "SmithPredictor"
  Yp/1 -> Scope1/1, Sum17/2  "SmithPredictor"
  LTI System16/1 -> LTI System17/1, Sum18/1
  Sum18/1 -> Sum/2
  LTI System17/1 -> Scope1/2, Sum17/1
  Sum17/1 -> Sum18/2
  theta/1 -> Mul/2, Scope/1
  Rate Limiter3/1 -> LTI System16/1, U/1

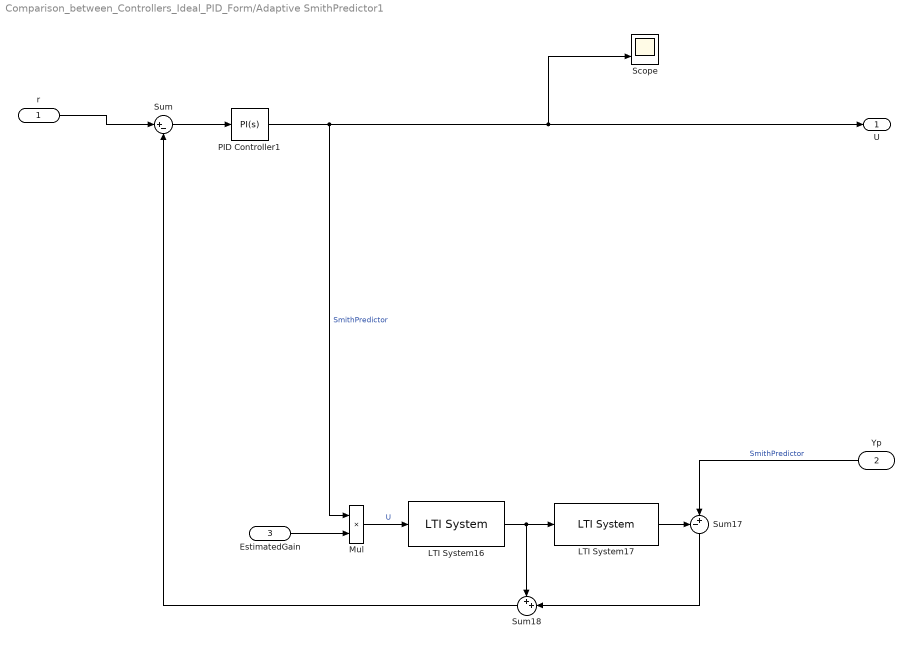
== system Comparison_between_Controllers_Ideal_PID_Form/Adaptive SmithPredictor1 ==
  r : Inport
  Yp : Inport  Port=2
  EstimatedGain : Inport  Port=3
  LTI System16 : cstblocks/LTI System  sys=1/(700*s+1)  IC=[]
  LTI System17 : cstblocks/LTI System  sys=exp(-s*600)  IC=[]
  Mul : Product
  PID Controller1 : simulink/Continuous/PID Controller  Controller=PI  Form=Parallel  TimeDomain=Continuous-time  SampleTime=-1  IntegratorMethod=Forward Euler  FilterMethod=Forward Euler  ControllerParametersSource=internal  P=3.04732259067536  I=0.00445689106465138  D=118.272348286844  UseFilter=on  N=0.00420306193364532  TunerSelectOption=Transfer Function Based (PID Tuner App)  InitialConditionSource=internal  InitialConditionForIntegrator=0  InitialConditionForFilter=0  DifferentiatorICPrevScaledInput=0  ExternalReset=none  TrackingMode=off  Kt=1  LimitOutput=on  UpperSaturationLimit=100  LowerSaturationLimit=0  LinearizeAsGain=on  AntiWindupMode=none  Kb=1  POutMin=[]  POutMax=[]  IOutMin=[]  IOutMax=[]  DOutMin=[]  DOutMax=[]  NOutMin=[]  NOutMax=[]  SumOutMin=[]  SumOutMax=[]  SaturationOutMin=[]  SaturationOutMax=[]  PParamMin=[]  PParamMax=[]  IParamMin=[]  IParamMax=[]  DParamMin=[]  DParamMax=[]  NParamMin=[]  NParamMax=[]  KbParamMin=[]  KbParamMax=[]  KtParamMin=[]  KtParamMax=[]  KbOutMin=[]  KbOutMax=[]  KtOutMin=[]  KtOutMax=[]  IntegratorOutMin=[]  IntegratorOutMax=[]  FilterOutMin=[]  FilterOutMax=[]  SumI1OutMin=[]  SumI1OutMax=[]  SumI2OutMin=[]  SumI2OutMax=[]  SumI3OutMin=[]  SumI3OutMax=[]  SumI4OutMin=[]  SumI4OutMax=[]  SumDOutMin=[]  SumDOutMax=[]  DifferentiatorOutMin=[]  DifferentiatorOutMax=[]  FilterDiffOutCoefMin=[]  FilterDiffOutCoefMax=[]  ReciprocalOutMin=[]  ReciprocalOutMax=[]  SumDenOutMin=[]  SumDenOutMax=[]  SumNumOutMin=[]  SumNumOutMax=[]  DivideOutMin=[]  DivideOutMax=[]  IntegratorContinuousStateAttributes=''  IntegratorStateMustResolveToSignalObject=off  IntegratorRTWStateStorageClass=Auto  FilterContinuousStateAttributes=''  FilterStateMustResolveToSignalObject=off  FilterRTWStateStorageClass=Auto  ParallelPVariant=InternalParameters  IdealPVariant=Disabled  IVariant=InternalParameters  DVariant=Disabled  IntegratorVariant=Continuous  SatVariant=Enabled  AWVariant=Passthrough  PCopyVariant=Disabled  TRVariant=Disabled  FdbkBlocksVariant=Forward  IdealPFdbkVariant=Disabled  SatFdbkVariant=Disabled  DerivativeFilterVariant=Disabled  NVariant=Disabled  NCopyVariant=Disabled_SignalSpec  FilterICVariant=Disabled  IntegratorICVariant=InternalICs  ExternalResetVariant=Disabled  TRSumVariant=Passthrough  SumFdbkVariant=Disabled  SumVariant=Sum_PI
  Scope : Scope  NumInputPorts=2
  Sum : Sum  Inputs=|+-
  Sum17 : Sum  Inputs=-+|
  Sum18 : Sum  Inputs=++|
  U : Outport
  wires:
  r/1 -> Sum/1
  Sum/1 -> PID Controller1/1
  PID Controller1/1 -> Scope/2, U/1, Mul/1  "SmithPredictor"
  Yp/1 -> Sum17/2  "SmithPredictor"
  LTI System16/1 -> LTI System17/1, Sum18/1
  Sum18/1 -> Sum/2
  LTI System17/1 -> Sum17/1
  Sum17/1 -> Sum18/2
  Mul/1 -> LTI System16/1  "U"
  EstimatedGain/1 -> Mul/2

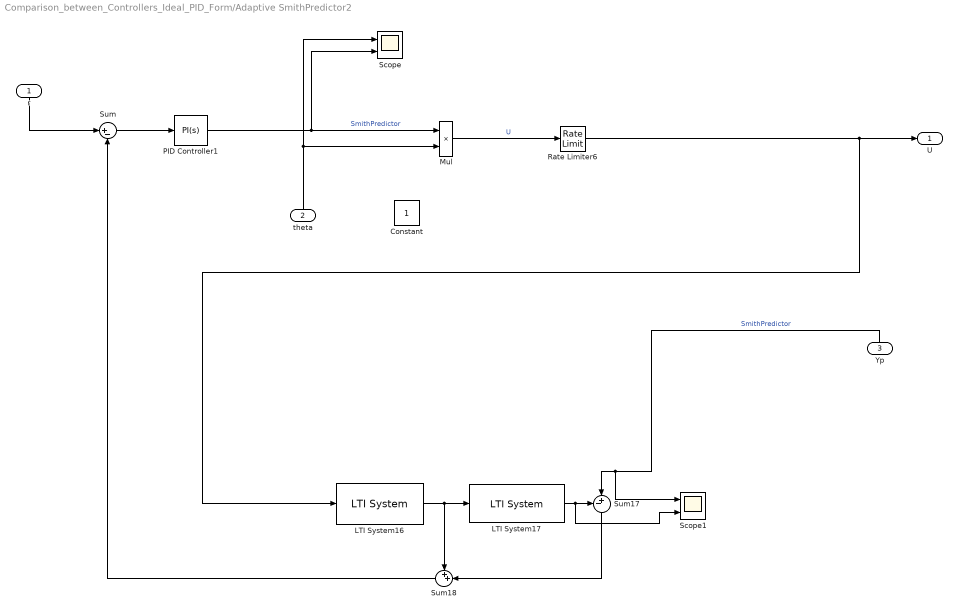
== system Comparison_between_Controllers_Ideal_PID_Form/Adaptive SmithPredictor2 ==
  r : Inport
  theta : Inport  Port=2
  Yp : Inport  Port=3
  Constant : Constant
  LTI System16 : cstblocks/LTI System  sys=0.5/(700*s+1)  IC=[]
  LTI System17 : cstblocks/LTI System  sys=exp(-s*600)  IC=[]
  Mul : Product
  PID Controller1 : simulink/Continuous/PID Controller  Controller=PI  Form=Parallel  TimeDomain=Continuous-time  SampleTime=-1  IntegratorMethod=Forward Euler  FilterMethod=Forward Euler  ControllerParametersSource=internal  P=3.04732259067536  I=0.00445689106465138  D=118.272348286844  UseFilter=on  N=0.00420306193364532  TunerSelectOption=Transfer Function Based (PID Tuner App)  InitialConditionSource=internal  InitialConditionForIntegrator=0  InitialConditionForFilter=0  DifferentiatorICPrevScaledInput=0  ExternalReset=none  TrackingMode=off  Kt=1  LimitOutput=on  UpperSaturationLimit=100  LowerSaturationLimit=0  LinearizeAsGain=on  AntiWindupMode=none  Kb=1  POutMin=[]  POutMax=[]  IOutMin=[]  IOutMax=[]  DOutMin=[]  DOutMax=[]  NOutMin=[]  NOutMax=[]  SumOutMin=[]  SumOutMax=[]  SaturationOutMin=[]  SaturationOutMax=[]  PParamMin=[]  PParamMax=[]  IParamMin=[]  IParamMax=[]  DParamMin=[]  DParamMax=[]  NParamMin=[]  NParamMax=[]  KbParamMin=[]  KbParamMax=[]  KtParamMin=[]  KtParamMax=[]  KbOutMin=[]  KbOutMax=[]  KtOutMin=[]  KtOutMax=[]  IntegratorOutMin=[]  IntegratorOutMax=[]  FilterOutMin=[]  FilterOutMax=[]  SumI1OutMin=[]  SumI1OutMax=[]  SumI2OutMin=[]  SumI2OutMax=[]  SumI3OutMin=[]  SumI3OutMax=[]  SumI4OutMin=[]  SumI4OutMax=[]  SumDOutMin=[]  SumDOutMax=[]  DifferentiatorOutMin=[]  DifferentiatorOutMax=[]  FilterDiffOutCoefMin=[]  FilterDiffOutCoefMax=[]  ReciprocalOutMin=[]  ReciprocalOutMax=[]  SumDenOutMin=[]  SumDenOutMax=[]  SumNumOutMin=[]  SumNumOutMax=[]  DivideOutMin=[]  DivideOutMax=[]  IntegratorContinuousStateAttributes=''  IntegratorStateMustResolveToSignalObject=off  IntegratorRTWStateStorageClass=Auto  FilterContinuousStateAttributes=''  FilterStateMustResolveToSignalObject=off  FilterRTWStateStorageClass=Auto  ParallelPVariant=InternalParameters  IdealPVariant=Disabled  IVariant=InternalParameters  DVariant=Disabled  IntegratorVariant=Continuous  SatVariant=Enabled  AWVariant=Passthrough  PCopyVariant=Disabled  TRVariant=Disabled  FdbkBlocksVariant=Forward  IdealPFdbkVariant=Disabled  SatFdbkVariant=Disabled  DerivativeFilterVariant=Disabled  NVariant=Disabled  NCopyVariant=Disabled_SignalSpec  FilterICVariant=Disabled  IntegratorICVariant=InternalICs  ExternalResetVariant=Disabled  TRSumVariant=Passthrough  SumFdbkVariant=Disabled  SumVariant=Sum_PI
  Rate Limiter6 : RateLimiter  RisingSlewLimit=0.05  FallingSlewLimit=-0.05  SampleTimeMode=inherited
  Scope : Scope  NumInputPorts=2
  Scope1 : Scope  NumInputPorts=2
  Sum : Sum  Inputs=|+-
  Sum17 : Sum  Inputs=-+|
  Sum18 : Sum  Inputs=++|
  U : Outport
  wires:
  r/1 -> Sum/1
  Sum/1 -> PID Controller1/1
  Mul/1 -> Rate Limiter6/1  "U"
  PID Controller1/1 -> Scope/2, Mul/1  "SmithPredictor"
  Yp/1 -> Scope1/1, Sum17/2  "SmithPredictor"
  LTI System16/1 -> LTI System17/1, Sum18/1
  Sum18/1 -> Sum/2
  LTI System17/1 -> Scope1/2, Sum17/1
  Sum17/1 -> Sum18/2
  theta/1 -> Mul/2, Scope/1
  Rate Limiter6/1 -> LTI System16/1, U/1

== system Comparison_between_Controllers_Ideal_PID_Form/Calculate DC Gain ==
  Params : Inport
  A(z) Sum of Elements : Sum  Inputs=+
  B(z) Sum of Elements : Sum  Inputs=+
  Bus Selector : BusSelector  OutputSignals=B,A
  Divide : Product  Inputs=*/
  DCGain : Outport
  wires:
  A(z) Sum of Elements/1 -> Divide/2
  B(z) Sum of Elements/1 -> Divide/1
  Params/1 -> Bus Selector/1
  Bus Selector/1 -> B(z) Sum of Elements/1  "<B>"
  Bus Selector/2 -> A(z) Sum of Elements/1  "<A>"
  Divide/1 -> DCGain/1  "DCGain"

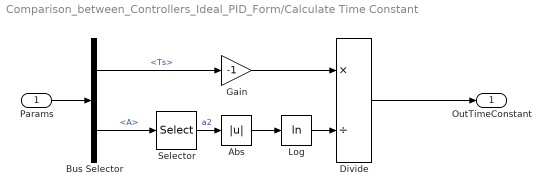
== system Comparison_between_Controllers_Ideal_PID_Form/Calculate Time Constant ==
  Params : Inport
  Abs : Abs
  Bus Selector : BusSelector  OutputSignals=Ts,A
  Divide : Product  Inputs=*/
  Gain : Gain  Gain=-1
  Log : Math  Operator=log  SaturateOnIntegerOverflow=on
  Selector : Selector  InputPortWidth=2  IndexOptions=Starting index (dialog)  Indices=[2]  OutputSizes=1
  "OutTimeConstant " : Outport
  wires:
  Params/1 -> Bus Selector/1
  Bus Selector/1 -> Gain/1  "<Ts>"
  Bus Selector/2 -> Selector/1  "<A>"
  Selector/1 -> Abs/1  "a2"
  Gain/1 -> Divide/1
  Log/1 -> Divide/2
  Divide/1 -> "OutTimeConstant "/1
  Abs/1 -> Log/1

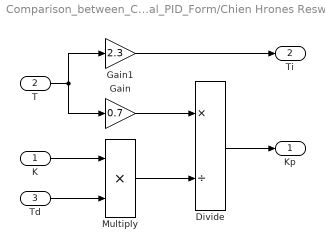
== system Comparison_between_Controllers_Ideal_PID_Form/Chien Hrones Reswick ==
  K : Inport
  T : Inport  Port=2
  Td : Inport  Port=3
  Divide : Product  Inputs=*/
  Gain : Gain  Gain=0.7
  Gain1 : Gain  Gain=2.3
  Multiply : Product
  Kp : Outport
  Ti : Outport  Port=2
  wires:
  T/1 -> Gain/1, Gain1/1
  Gain/1 -> Divide/1
  Td/1 -> Multiply/2
  Multiply/1 -> Divide/2
  Divide/1 -> Kp/1
  K/1 -> Multiply/1
  Gain1/1 -> Ti/1

== system Comparison_between_Controllers_Ideal_PID_Form/Reference_Model ==
  r : Inport
  Transfer_Function2 : TransferFcn  Denominator=[450 1]
  Transport Delay2 : TransportDelay  DelayTime=600
  Ym : Outport
  wires:
  Transfer_Function2/1 -> Transport Delay2/1  "Ym"
  r/1 -> Transfer_Function2/1
  Transport Delay2/1 -> Ym/1  "Adaptive_Plant"

== system Comparison_between_Controllers_Ideal_PID_Form/Reference_Model1 ==
  r : Inport
  Transfer_Function2 : TransferFcn  Denominator=[450 1]
  Ym : Outport
  wires:
  Transfer_Function2/1 -> Ym/1  "Ym"
  r/1 -> Transfer_Function2/1

== system Comparison_between_Controllers_Ideal_PID_Form/Reference_Model2 ==
  r : Inport
  Transfer_Function2 : TransferFcn  Denominator=[450 1]
  Transport Delay2 : TransportDelay  DelayTime=600
  Ym : Outport
  wires:
  Transfer_Function2/1 -> Transport Delay2/1  "Ym"
  r/1 -> Transfer_Function2/1
  Transport Delay2/1 -> Ym/1  "Adaptive_Plant"

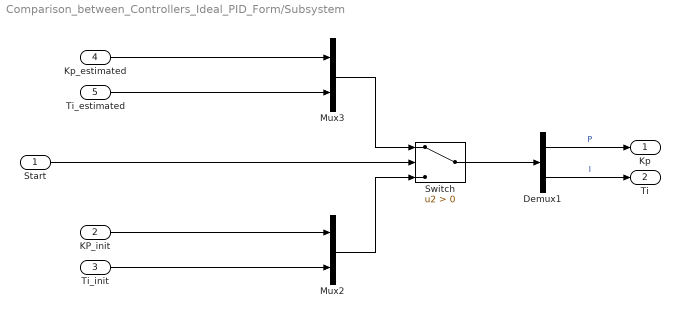
== system Comparison_between_Controllers_Ideal_PID_Form/Subsystem ==
  Start : Inport
  KP_init : Inport  Port=2
  Ti_init : Inport  Port=3
  Kp_estimated : Inport  Port=4
  Ti_estimated : Inport  Port=5
  Demux1 : Demux  Outputs=2
  Mux2 : Mux  Inputs=2
  Mux3 : Mux  Inputs=2
  Switch : Switch  Criteria=u2 > Threshold
  Kp : Outport
  Ti : Outport  Port=2
  wires:
  Mux3/1 -> Switch/1
  Mux2/1 -> Switch/3
  Start/1 -> Switch/2
  Switch/1 -> Demux1/1
  KP_init/1 -> Mux2/1
  Ti_init/1 -> Mux2/2
  Kp_estimated/1 -> Mux3/1
  Ti_estimated/1 -> Mux3/2
  Demux1/1 -> Kp/1  "P"
  Demux1/2 -> Ti/1  "I"

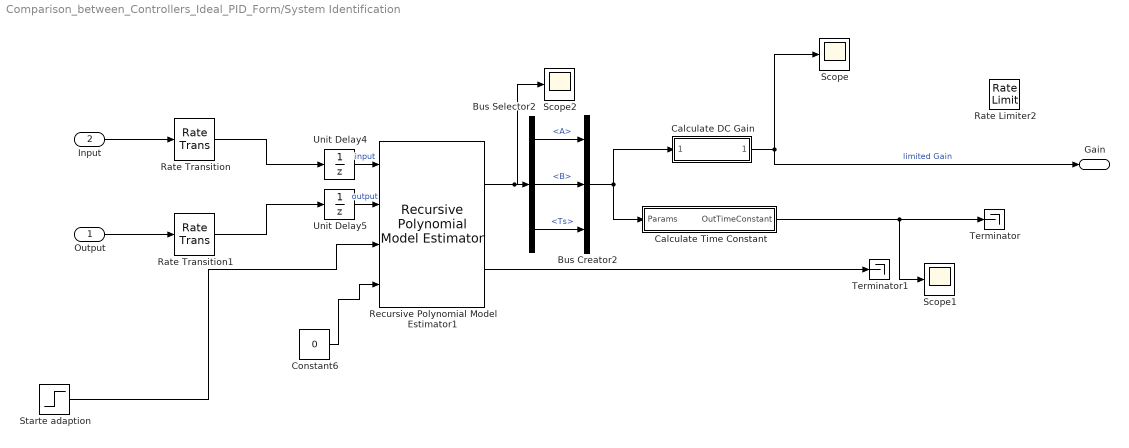
== system Comparison_between_Controllers_Ideal_PID_Form/System Identification ==
  Output : Inport
  Input : Inport  Port=2
  Bus Creator2 : BusCreator  Inputs=3
  Bus Selector2 : BusSelector  OutputSignals=A,B,Ts
  Calculate DC Gain : Subsystem
  Calculate Time Constant : Subsystem
  Constant6 : Constant  Value=0  SampleTime=1
  Rate Limiter2 : RateLimiter  SampleTimeMode=inherited
  Rate Transition : RateTransition  OutPortSampleTime=1
  Rate Transition1 : RateTransition  OutPortSampleTime=1
  Recursive Polynomial Model Estimator1 : slident/Estimators/Recursive Polynomial Model Estimator  ModelStructure=ARX  InitialEstimateSource=None  A0=1  B0=1  C0=1  D0=1  F0=1  nk=1  P0=1  InitialInputs=0  InitialOutputs=0  History=Infinite  WindowLength=2000  EstimationMethod=Forgetting Factor  AdaptationParameter=1  HasTimeVaryingAdaptationParameter=off  NormalizationBias=eps  OutputError=on  OutputP=off  AddEnablePort=on  ExternalReset=Rising  InputProcessing=Sample-based  Ts=1
      settings: SourceProductName=System Identification Toolbox  SourceProductBaseCode=ID
  Scope : Scope
  Scope1 : Scope
  Scope2 : Scope
  Starte adaption : Step  Time=0  SampleTime=1
  Terminator : Terminator
  Terminator1 : Terminator
  Unit Delay4 : UnitDelay  InitialCondition=[0]
  Unit Delay5 : UnitDelay
  Gain : Outport
  wires:
  Bus Selector2/1 -> Bus Creator2/1  "<A>"
  Recursive Polynomial Model Estimator1/1 -> Scope2/1, Bus Selector2/1
  Bus Selector2/3 -> Bus Creator2/3  "<Ts>"
  Bus Selector2/2 -> Bus Creator2/2  "<B>"
  Bus Creator2/1 -> Calculate DC Gain/1(Params), Calculate Time Constant/1(Params)
  Recursive Polynomial Model Estimator1/2 -> Terminator1/1
  Calculate DC Gain/1(DCGain) -> Gain/1, Scope/1  "limited Gain"
  Calculate Time Constant/1("OutTimeConstant ") -> Scope1/1, Terminator/1
  Constant6/1 -> Recursive Polynomial Model Estimator1/4
  Unit Delay4/1 -> Recursive Polynomial Model Estimator1/1  "input"
  Unit Delay5/1 -> Recursive Polynomial Model Estimator1/2  "output"
  Input/1 -> Rate Transition/1
  Output/1 -> Rate Transition1/1
  Rate Transition/1 -> Unit Delay4/1
  Rate Transition1/1 -> Unit Delay5/1
  Starte adaption/1 -> Recursive Polynomial Model Estimator1/3
